simulink model "BallAndBeam_function"  (R2020b)
settings: Solver=ode4  StartTime=0.0  StopTime=10.0  FixedStep=0.01  RelTol=1e-3
libraries: fuzblock x1
settings Model: Creator=Long  LastModifiedBy=Long

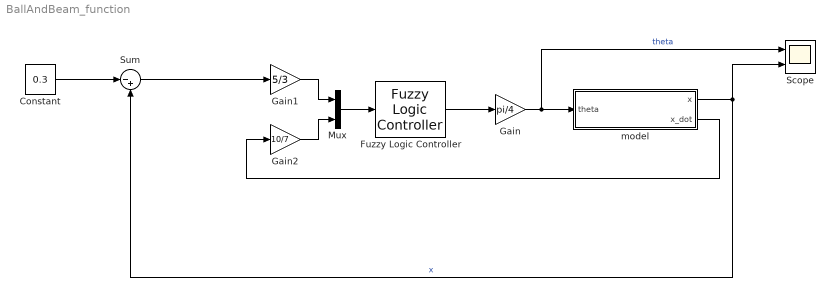
== system BallAndBeam_function ==
  Constant : Constant  Value=0.3
  Fuzzy Logic Controller : fuzblock/Fuzzy Logic  Controller  FIS='BallAndBeam_FuzzyController.fis'  OutputSampleNumber=101  DataType=double  FuzzifiedInputs=off  RuleFiringStrengths=off  RuleOutputs=off  AggregatedOutputs=off  SimulateUsing=Interpreted execution  OutOfRangeInputValueMessage=warning  NoRuleFiredMessage=warning  EmptyOutputFuzzySetMessage=warning
  Gain : Gain  Gain=pi/4
  Gain1 : Gain  Gain=5/3
  Gain2 : Gain  Gain=10/7
  Mux : Mux  Inputs=2
  Scope : Scope  NumInputPorts=2
  Sum : Sum  Inputs=|-+
  model : Subsystem  mask{x0=-0.2}
  wires:
  Fuzzy Logic Controller/1 -> Gain/1
  Gain/1 -> Scope/1, model/1(theta)  "theta"
  Gain1/1 -> Mux/1
  Gain2/1 -> Mux/2
  Mux/1 -> Fuzzy Logic Controller/1
  model/1(x) -> Scope/2, Sum/2  "x"
  model/2(x_dot) -> Gain2/1
  Constant/1 -> Sum/1
  Sum/1 -> Gain1/1

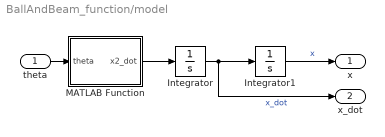
== system BallAndBeam_function/model ==
  theta : Inport
  Integrator : Integrator
  Integrator1 : Integrator  InitialCondition=x0
  MATLAB Function : MATLAB Function  TreatAsAtomicUnit=on
  x : Outport
  x_dot : Outport  Port=2
  wires:
  MATLAB Function/1(x2_dot) -> Integrator/1
  Integrator1/1 -> x/1  "x"
  Integrator/1 -> x_dot/1, Integrator1/1  "x_dot"
  theta/1 -> MATLAB Function/1(theta)

== matlab function BallAndBeam_function/model/MATLAB Function ==
  data: theta input; x2_dot output
function x2_dot = fcn(theta)
%% model parameters
m = 1;
J = 3.3e-5;
R = 5e-3;
g =9.81;
%%

x2_dot = (m*g*sin(theta))/((J/R^2)+m);
